simulink model "Robo_Bipede_Contato"  (R2020a)
settings: Solver=ode15s  StartTime=0.0  StopTime=ts  MaxStep=1e-4  RelTol=1e-4  AbsTol=1e-5  EnableMultiTasking=on
model workspace: external: MATLAB File C:\Users\LUIS IZQUIERDO C\Desktop\PROGRAMAS TESE\13. ROBO BIPEDE SIMSCAPE COM CONTATO\Model_Params_Contato.m (data not in the file)
values from neighbouring files (symbols this model uses):
  CoG_y = 0.091733    [Model_Params_Contato.m]
  height_plane = 0.025    [Model_Params_Contato.m]
  m_esfera = 1    [Model_Params_Contato.m]
  plane_height = height_plane    (= 0.025)    [Model_Params_Contato.m]
  plane_length = 50    [Model_Params_Contato.m]
  plane_width = 3    [Model_Params_Contato.m]
  velocidade = 3    [Model_Params_Contato.m]
undefined symbols (not defined in the file or in its folder): COXA, HAT, PE, PERNA, X, Y, Z
libraries: nesl_utility x70, sm_lib x61, simulink_extras x2, simulink x1
(part 2 of 2)

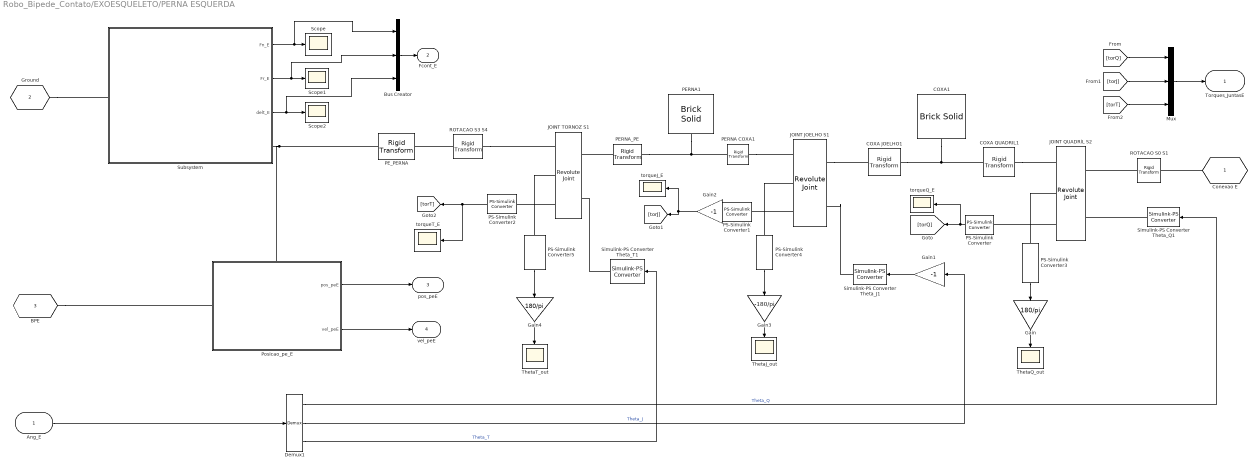
== system Robo_Bipede_Contato/EXOESQUELETO/PERNA ESQUERDA ==
  Ang_E : Inport
  Bus Creator : BusCreator  Inputs=3
  COXA JOELHO1 : sm_lib/Frames and Transforms/Rigid Transform  TranslationMethod=StandardAxis  TranslationStandardOffset=COXA.Comprimento/2  TranslationLengthUnit=m  TranslationStandardAxis=+X  TranslationCartesianOffset=[0 0 0]  TranslationROffset=0  TranslationROffsetUnits=m  TranslationZOffset=0  TranslationZOffsetUnits=m  TranslationThetaOffset=0  TranslationThetaOffsetUnits=deg  RotationMethod=None  RotationAngleUnits=deg  RotationStandardAxis=+Z  RotationAngle=0.0  RotationArbitraryAxis=[0 0 1]  FollAlignAxisA=+X  BaseAlignAxisA=+Y  FollAlignAxisB=+Y  BaseAlignAxisB=+Z  RotationSequenceAxes=FollowerAxes  RotationSequence=XYX  RotationSequenceAngles=[0 0 0]  RotationSequenceAnglesUnits=deg  RotationMatrix=[1 0 0; 0 1 0; 0 0 1]
  COXA QUADRIL1 : sm_lib/Frames and Transforms/Rigid Transform  TranslationMethod=StandardAxis  TranslationStandardOffset=COXA.Comprimento/2  TranslationLengthUnit=m  TranslationStandardAxis=-X  TranslationCartesianOffset=[0 0 0]  TranslationROffset=0  TranslationROffsetUnits=m  TranslationZOffset=0  TranslationZOffsetUnits=m  TranslationThetaOffset=0  TranslationThetaOffsetUnits=deg  RotationMethod=None  RotationAngleUnits=deg  RotationStandardAxis=+Z  RotationAngle=0.0  RotationArbitraryAxis=[0 0 1]  FollAlignAxisA=+X  BaseAlignAxisA=+Y  FollAlignAxisB=+Y  BaseAlignAxisB=+Z  RotationSequenceAxes=FollowerAxes  RotationSequence=XYX  RotationSequenceAngles=[0 0 0]  RotationSequenceAnglesUnits=deg  RotationMatrix=[1 0 0; 0 1 0; 0 0 1]
  COXA1 : sm_lib/Body Elements/Brick Solid  GraphicAmbientColor=[0.15 0.15 0.15 1.0]  BasedOnType=Density  BrickDimensions="[COXA.Comprimento,  COXA.Profundidade,  COXA.Largura]"  BrickDimensionUnits=m  CenterOfMass=[0 0 0]  CenterOfMassUnits=m  GraphicDiffuseColor=cor_coxa  Density=rho_ABS  DensityUnits=kg/m^3  DoExposeReferenceFrame=on  GraphicEmissiveColor=[0.0 0.0 0.0 1.0]  ExportEntireGeometry=off  SerializedFrames=<Frames/>  MarkerShape=Sphere  MarkerSize=10  GraphicType=FromGeometry  InertiaType=CalculateFromGeometry  Mass=1  MassUnits=kg  MomentsOfInertia=[1 1 1]  MomentsOfInertiaUnits=kg*m^2  GraphicOpacity=1.0  ProductsOfInertia=[0 0 0]  ProductsOfInertiaUnits=kg*m^2  GraphicShininess=75  GraphicSpecularColor=[0.5 0.5 0.5 1.0]  GraphicVisPropType=SimpleVisualProperties
  Demux1 : Demux  Outputs=3
  Gain : Gain  Gain=180/pi
  Gain1 : Gain  Gain=-1
  Gain2 : Gain  Gain=-1
  Gain3 : Gain  Gain=-180/pi
  Gain4 : Gain  Gain=180/pi
  JOINT JOELHO S1 : sm_lib/Joints/Revolute Joint  JointMode=Normal  SenseConstraintForce=off  SenseConstraintForceX=off  SenseConstraintForceY=off  SenseConstraintForceZ=off  SenseConstraintTorque=off  SenseConstraintTorqueX=off  SenseConstraintTorqueY=off  SenseConstraintTorqueZ=off  SenseTotalForce=off  SenseTotalForceX=off  SenseTotalForceY=off  SenseTotalForceZ=off  SenseTotalTorque=off  SenseTotalTorqueX=off  SenseTotalTorqueY=off  SenseTotalTorqueZ=off  CompositeWrenchDir=FollowerOnBase  CompositeWrenchFrame=BaseFrame  EquilibriumPosition=0  EquilibriumPositionUnits=rad  SpringStiffness=0  SpringStiffnessUnits=N*m/rad  DampingCoefficient=Damping_junta  DampingCoefficientUnits=N*m/(rad/s)  TorqueActuationMode=ComputedTorque  MotionActuationMode=InputMotion  SensePosition=on  SenseVelocity=off  SenseAcceleration=off  SenseTorqueForce=on  SenseLowerLimitTorqueForce=off  SenseUpperLimitTorqueForce=off  LowerLimitSpecify=off  LowerLimitBound=-90  LowerLimitBoundUnits=deg  LowerLimitStiffness=1e4  LowerLimitStiffnessUnits=N*m/deg  LowerLimitDamping=10  LowerLimitDampingUnits=N*m/(deg/s)  LowerLimitTransitionRegionWidth=0.1  LowerLimitTransitionRegionWidthUnits=deg  UpperLimitSpecify=off  UpperLimitBound=90  UpperLimitBoundUnits=deg  UpperLimitStiffness=1e4  UpperLimitStiffnessUnits=N*m/deg  UpperLimitDamping=10  UpperLimitDampingUnits=N*m/(deg/s)  UpperLimitTransitionRegionWidth=0.1  UpperLimitTransitionRegionWidthUnits=deg  PositionTargetSpecify=on  PositionTargetPriority=High  PositionTargetValue=thetaJ_E0  PositionTargetValueUnits=rad  VelocityTargetSpecify=off  VelocityTargetPriority=High  VelocityTargetValue=0  VelocityTargetValueUnits=deg/s
  JOINT QUADRlL S2 : sm_lib/Joints/Revolute Joint  JointMode=Normal  SenseConstraintForce=off  SenseConstraintForceX=off  SenseConstraintForceY=off  SenseConstraintForceZ=off  SenseConstraintTorque=off  SenseConstraintTorqueX=off  SenseConstraintTorqueY=off  SenseConstraintTorqueZ=off  SenseTotalForce=off  SenseTotalForceX=off  SenseTotalForceY=off  SenseTotalForceZ=off  SenseTotalTorque=off  SenseTotalTorqueX=off  SenseTotalTorqueY=off  SenseTotalTorqueZ=off  CompositeWrenchDir=FollowerOnBase  CompositeWrenchFrame=BaseFrame  EquilibriumPosition=0  EquilibriumPositionUnits=rad  SpringStiffness=0  SpringStiffnessUnits=N*m/rad  DampingCoefficient=Damping_junta  DampingCoefficientUnits=N*m/(rad/s)  TorqueActuationMode=ComputedTorque  MotionActuationMode=InputMotion  SensePosition=on  SenseVelocity=off  SenseAcceleration=off  SenseTorqueForce=on  SenseLowerLimitTorqueForce=off  SenseUpperLimitTorqueForce=off  LowerLimitSpecify=off  LowerLimitBound=-90  LowerLimitBoundUnits=deg  LowerLimitStiffness=1e4  LowerLimitStiffnessUnits=N*m/deg  LowerLimitDamping=10  LowerLimitDampingUnits=N*m/(deg/s)  LowerLimitTransitionRegionWidth=0.1  LowerLimitTransitionRegionWidthUnits=deg  UpperLimitSpecify=off  UpperLimitBound=90  UpperLimitBoundUnits=deg  UpperLimitStiffness=1e4  UpperLimitStiffnessUnits=N*m/deg  UpperLimitDamping=10  UpperLimitDampingUnits=N*m/(deg/s)  UpperLimitTransitionRegionWidth=0.1  UpperLimitTransitionRegionWidthUnits=deg  PositionTargetSpecify=on  PositionTargetPriority=High  PositionTargetValue=thetaQ_E0  PositionTargetValueUnits=rad  VelocityTargetSpecify=off  VelocityTargetPriority=High  VelocityTargetValue=0  VelocityTargetValueUnits=deg/s
  JOINT TORNOZ S1 : sm_lib/Joints/Revolute Joint  JointMode=Normal  SenseConstraintForce=off  SenseConstraintForceX=off  SenseConstraintForceY=off  SenseConstraintForceZ=off  SenseConstraintTorque=off  SenseConstraintTorqueX=off  SenseConstraintTorqueY=off  SenseConstraintTorqueZ=off  SenseTotalForce=off  SenseTotalForceX=off  SenseTotalForceY=off  SenseTotalForceZ=off  SenseTotalTorque=off  SenseTotalTorqueX=off  SenseTotalTorqueY=off  SenseTotalTorqueZ=off  CompositeWrenchDir=FollowerOnBase  CompositeWrenchFrame=BaseFrame  EquilibriumPosition=0  EquilibriumPositionUnits=rad  SpringStiffness=0  SpringStiffnessUnits=N*m/rad  DampingCoefficient=Damping_junta  DampingCoefficientUnits=N*m/(rad/s)  TorqueActuationMode=ComputedTorque  MotionActuationMode=InputMotion  SensePosition=on  SenseVelocity=off  SenseAcceleration=off  SenseTorqueForce=on  SenseLowerLimitTorqueForce=off  SenseUpperLimitTorqueForce=off  LowerLimitSpecify=off  LowerLimitBound=-90  LowerLimitBoundUnits=deg  LowerLimitStiffness=1e4  LowerLimitStiffnessUnits=N*m/deg  LowerLimitDamping=10  LowerLimitDampingUnits=N*m/(deg/s)  LowerLimitTransitionRegionWidth=0.1  LowerLimitTransitionRegionWidthUnits=deg  UpperLimitSpecify=off  UpperLimitBound=90  UpperLimitBoundUnits=deg  UpperLimitStiffness=1e4  UpperLimitStiffnessUnits=N*m/deg  UpperLimitDamping=10  UpperLimitDampingUnits=N*m/(deg/s)  UpperLimitTransitionRegionWidth=0.1  UpperLimitTransitionRegionWidthUnits=deg  PositionTargetSpecify=on  PositionTargetPriority=High  PositionTargetValue=thetaT_E0  PositionTargetValueUnits=rad  VelocityTargetSpecify=off  VelocityTargetPriority=High  VelocityTargetValue=0  VelocityTargetValueUnits=deg/s
  Mux : Mux  Inputs=3
  PERNA COXA1 : sm_lib/Frames and Transforms/Rigid Transform  TranslationMethod=StandardAxis  TranslationStandardOffset=PERNA.Comprimento/2  TranslationLengthUnit=m  TranslationStandardAxis=-X  TranslationCartesianOffset=[0 0 0]  TranslationROffset=0  TranslationROffsetUnits=m  TranslationZOffset=0  TranslationZOffsetUnits=m  TranslationThetaOffset=0  TranslationThetaOffsetUnits=deg  RotationMethod=None  RotationAngleUnits=deg  RotationStandardAxis=+Z  RotationAngle=0.0  RotationArbitraryAxis=[0 0 1]  FollAlignAxisA=+X  BaseAlignAxisA=+Y  FollAlignAxisB=+Y  BaseAlignAxisB=+Z  RotationSequenceAxes=FollowerAxes  RotationSequence=XYX  RotationSequenceAngles=[0 0 0]  RotationSequenceAnglesUnits=deg  RotationMatrix=[1 0 0; 0 1 0; 0 0 1]
  PERNA1 : sm_lib/Body Elements/Brick Solid  GraphicAmbientColor=[0.15 0.15 0.15 1.0]  BasedOnType=Density  BrickDimensions=[PERNA.Comprimento, PERNA.Profundidade, PERNA.Largura]  BrickDimensionUnits=m  CenterOfMass=[0 0 0]  CenterOfMassUnits=m  GraphicDiffuseColor=cor_perna  Density=rho_ABS  DensityUnits=kg/m^3  DoExposeReferenceFrame=on  GraphicEmissiveColor=[0.0 0.0 0.0 1.0]  ExportEntireGeometry=off  SerializedFrames=<Frames/>  MarkerShape=Sphere  MarkerSize=10  GraphicType=FromGeometry  InertiaType=CalculateFromGeometry  Mass=1  MassUnits=kg  MomentsOfInertia=[1 1 1]  MomentsOfInertiaUnits=kg*m^2  GraphicOpacity=1.0  ProductsOfInertia=[0 0 0]  ProductsOfInertiaUnits=kg*m^2  GraphicShininess=75  GraphicSpecularColor=[0.5 0.5 0.5 1.0]  GraphicVisPropType=SimpleVisualProperties
  PERNA_PE : sm_lib/Frames and Transforms/Rigid Transform  TranslationMethod=Cartesian  TranslationStandardOffset=0  TranslationLengthUnit=m  TranslationStandardAxis=+Z  TranslationCartesianOffset=[PERNA.Comprimento/2, -PERNA.Profundidade/2, 0]  TranslationROffset=0  TranslationROffsetUnits=m  TranslationZOffset=0  TranslationZOffsetUnits=m  TranslationThetaOffset=0  TranslationThetaOffsetUnits=deg  RotationMethod=None  RotationAngleUnits=deg  RotationStandardAxis=+Z  RotationAngle=0.0  RotationArbitraryAxis=[0 0 1]  FollAlignAxisA=+X  BaseAlignAxisA=+Y  FollAlignAxisB=+Y  BaseAlignAxisB=+Z  RotationSequenceAxes=FollowerAxes  RotationSequence=XYX  RotationSequenceAngles=[0 0 0]  RotationSequenceAnglesUnits=deg  RotationMatrix=[1 0 0; 0 1 0; 0 0 1]
  PE_PERNA : sm_lib/Frames and Transforms/Rigid Transform  TranslationMethod=Cartesian  TranslationStandardOffset=0  TranslationLengthUnit=m  TranslationStandardAxis=+Z  TranslationCartesianOffset=[-PE.Comprimento/2, 0, 0]  TranslationROffset=0  TranslationROffsetUnits=m  TranslationZOffset=0  TranslationZOffsetUnits=m  TranslationThetaOffset=0  TranslationThetaOffsetUnits=deg  RotationMethod=None  RotationAngleUnits=deg  RotationStandardAxis=+Z  RotationAngle=0.0  RotationArbitraryAxis=[0 0 1]  FollAlignAxisA=+X  BaseAlignAxisA=+Y  FollAlignAxisB=+Y  BaseAlignAxisB=+Z  RotationSequenceAxes=FollowerAxes  RotationSequence=XYX  RotationSequenceAngles=[0 0 0]  RotationSequenceAnglesUnits=deg  RotationMatrix=[1 0 0; 0 1 0; 0 0 1]
  PS-Simulink Converter : nesl_utility/PS-Simulink Converter  PhysicalDomain=network_engine_domain  SubClassName=ps_output  LeftPortType=input  RightPortType=output  PseudoPeriodic=off  Frequencies=[]  Unit=N*m  AffineConversion=off
  PS-Simulink Converter1 : nesl_utility/PS-Simulink Converter  PhysicalDomain=network_engine_domain  SubClassName=ps_output  LeftPortType=input  RightPortType=output  PseudoPeriodic=off  Frequencies=[]  Unit=N*m  AffineConversion=off
  PS-Simulink Converter2 : nesl_utility/PS-Simulink Converter  PhysicalDomain=network_engine_domain  SubClassName=ps_output  LeftPortType=input  RightPortType=output  PseudoPeriodic=off  Frequencies=[]  Unit=N*m  AffineConversion=off
  PS-Simulink Converter3 : nesl_utility/PS-Simulink Converter  PhysicalDomain=network_engine_domain  SubClassName=ps_output  LeftPortType=input  RightPortType=output  PseudoPeriodic=off  Frequencies=[]  Unit=1  AffineConversion=off
  PS-Simulink Converter4 : nesl_utility/PS-Simulink Converter  PhysicalDomain=network_engine_domain  SubClassName=ps_output  LeftPortType=input  RightPortType=output  PseudoPeriodic=off  Frequencies=[]  Unit=1  AffineConversion=off
  PS-Simulink Converter5 : nesl_utility/PS-Simulink Converter  PhysicalDomain=network_engine_domain  SubClassName=ps_output  LeftPortType=input  RightPortType=output  PseudoPeriodic=off  Frequencies=[]  Unit=1  AffineConversion=off
  Posicao_pe_E : Subsystem
      settings: PortSchema="{\"entries\":[{\"content\":{\"sides\":[{\"content\":{\"connectorIds\":[\"LConn1\"]},\"type\":\"ConnectorPlacement.EquallySpacedRectSide\",\"uuid\":\"d1ecfdf8-7ebe-4af1-bf63-6510536b3168\"},{\"content\":{\"connectorIds\":[\"Out1\",\"Out2\"],\"side\":\"RIGHT\"},\"type\":\"ConnectorPlacement.EquallySpacedRectSide\",\"uuid\":\"ea2203bb-aad8-4cc6-b714-1d05e8985fb0\"},{\"content\":{\"connectorIds\":[\"LConn2\"],\"side\":\"TOP\"},\"type\":\"ConnectorPlacement.EquallySpacedRectSide\",\"uuid\":\"9c93785d-a169-4ae6-a4ad-27289c508aaf\"}]},\"type\":\"ConnectorPlacement.EquallySpacedConnector\",\"uuid\":\"0aa9c047-7b9e-44d9-9c0d-089578f3a65a\"}],\"packageUris\":[\"http://schema.mathworks.com/mf0/Connector/19700101\"],\"version\":\"1.0\"}"
  ROTACAO S0 S1 : sm_lib/Frames and Transforms/Rigid Transform  TranslationMethod=None  TranslationStandardOffset=0  TranslationLengthUnit=m  TranslationStandardAxis=+Z  TranslationCartesianOffset=[0 0 0]  TranslationROffset=0  TranslationROffsetUnits=m  TranslationZOffset=0  TranslationZOffsetUnits=m  TranslationThetaOffset=0  TranslationThetaOffsetUnits=deg  RotationMethod=StandardAxis  RotationAngleUnits=deg  RotationStandardAxis=+Z  RotationAngle=-90  RotationArbitraryAxis=[0 0 1]  FollAlignAxisA=+X  BaseAlignAxisA=+Y  FollAlignAxisB=+Y  BaseAlignAxisB=+Z  RotationSequenceAxes=FollowerAxes  RotationSequence=XYX  RotationSequenceAngles=[0 0 0]  RotationSequenceAnglesUnits=deg  RotationMatrix=[1 0 0; 0 1 0; 0 0 1]
  ROTACAO S3 S4 : sm_lib/Frames and Transforms/Rigid Transform  TranslationMethod=None  TranslationStandardOffset=0  TranslationLengthUnit=m  TranslationStandardAxis=+Z  TranslationCartesianOffset=[0 0 0]  TranslationROffset=0  TranslationROffsetUnits=m  TranslationZOffset=0  TranslationZOffsetUnits=m  TranslationThetaOffset=0  TranslationThetaOffsetUnits=deg  RotationMethod=StandardAxis  RotationAngleUnits=deg  RotationStandardAxis=+Z  RotationAngle=90  RotationArbitraryAxis=[0 0 1]  FollAlignAxisA=+X  BaseAlignAxisA=+Y  FollAlignAxisB=+Y  BaseAlignAxisB=+Z  RotationSequenceAxes=FollowerAxes  RotationSequence=XYX  RotationSequenceAngles=[0 0 0]  RotationSequenceAnglesUnits=deg  RotationMatrix=[1 0 0; 0 1 0; 0 0 1]
  Scope : Scope
  Scope1 : Scope
  Scope2 : Scope
  Simulink-PS Converter Theta_J1 : nesl_utility/Simulink-PS Converter  PhysicalDomain=network_engine_domain  SubClassName=ps_input  LeftPortType=input  RightPortType=output  PseudoPeriodic=off  Frequencies=[]  NoiseDistribution=none  NoiseParameters=[]  Unit=rad  AffineConversion=off  FilteringAndDerivatives=filter  SimscapeFilterOrder=2  InputFilterTimeConstant=motion_time_constant  UdotUserProvided=0
  Simulink-PS Converter Theta_Q1 : nesl_utility/Simulink-PS Converter  PhysicalDomain=network_engine_domain  SubClassName=ps_input  LeftPortType=input  RightPortType=output  PseudoPeriodic=off  Frequencies=[]  NoiseDistribution=none  NoiseParameters=[]  Unit=rad  AffineConversion=off  FilteringAndDerivatives=filter  SimscapeFilterOrder=2  InputFilterTimeConstant=motion_time_constant  UdotUserProvided=0
  Simulink-PS Converter Theta_T1 : nesl_utility/Simulink-PS Converter  PhysicalDomain=network_engine_domain  SubClassName=ps_input  LeftPortType=input  RightPortType=output  PseudoPeriodic=off  Frequencies=[]  NoiseDistribution=none  NoiseParameters=[]  Unit=rad  AffineConversion=off  FilteringAndDerivatives=filter  SimscapeFilterOrder=2  InputFilterTimeConstant=motion_time_constant  UdotUserProvided=0
  Subsystem : Subsystem
  ThetaJ_out : Scope
  ThetaQ_out : Scope
  ThetaT_out : Scope
  torqueJ_E : Scope
  torqueQ_E : Scope
  torqueT_E : Scope
  Conexao E : PMIOPort  Side=Left
  Ground : PMIOPort  Port=2  Side=Left
  BPE : PMIOPort  Port=3  Side=Left
  "Torques_JuntasE " : Outport  VectorParamsAs1DForOutWhenUnconnected=off
  Fcont_E : Outport  Port=2
  pos_peE : Outport  Port=3
  vel_peE : Outport  Port=4
  wires:
  Gain2/1 -> torqueJ_E/1, [torJ]
  [torQ] -> Mux/1
  Mux/1 -> "Torques_JuntasE "/1
  [torT] -> Mux/3
  PS-Simulink Converter1/1 -> Gain2/1
  Ang_E/1 -> Demux1/1
  PS-Simulink Converter2/1 -> torqueT_E/1, [torT]
  PS-Simulink Converter/1 -> torqueQ_E/1, [torQ]
  Gain1/1 -> Simulink-PS Converter Theta_J1/1
  Demux1/1 -> Simulink-PS Converter Theta_Q1/1  "Theta_Q"
  Demux1/2 -> Gain1/1  "Theta_J"
  Demux1/3 -> Simulink-PS Converter Theta_T1/1  "Theta_T"
  [torJ] -> Mux/2
  Gain/1 -> ThetaQ_out/1
  PS-Simulink Converter3/1 -> Gain/1
  Gain3/1 -> ThetaJ_out/1
  PS-Simulink Converter4/1 -> Gain3/1
  PS-Simulink Converter5/1 -> Gain4/1
  Gain4/1 -> ThetaT_out/1
  Subsystem/3(delt_E) -> Bus Creator/3, Scope2/1
  Subsystem/2(Fr_E) -> Bus Creator/2, Scope1/1
  Subsystem/1(Fn_E) -> Bus Creator/1, Scope/1
  Bus Creator/1 -> Fcont_E/1
  Posicao_pe_E/1(pos_peE) -> pos_peE/1
  Posicao_pe_E/2(vel_peE) -> vel_peE/1
  connections:
  ROTACAO S3 S4/LConn1 -- JOINT TORNOZ S1/RConn1
  COXA JOELHO1/LConn1 -- COXA1/RConn1 -- COXA QUADRIL1/LConn1
  PERNA1/RConn1 -- PERNA COXA1/LConn1 -- PERNA_PE/LConn1
  ROTACAO S3 S4/RConn1 -- PE_PERNA/RConn1
  Simulink-PS Converter Theta_T1/RConn1 -- JOINT TORNOZ S1/LConn2
  PERNA COXA1/RConn1 -- JOINT JOELHO S1/RConn1
  Simulink-PS Converter Theta_Q1/RConn1 -- JOINT QUADRlL S2/LConn2
  JOINT JOELHO S1/LConn1 -- COXA JOELHO1/RConn1
  Simulink-PS Converter Theta_J1/RConn1 -- JOINT JOELHO S1/LConn2
  ROTACAO S0 S1/RConn1 -- JOINT QUADRlL S2/LConn1
  COXA QUADRIL1/RConn1 -- JOINT QUADRlL S2/RConn1
  Conexao E/RConn1 -- ROTACAO S0 S1/LConn1
  JOINT QUADRlL S2/RConn2 -- PS-Simulink Converter3/LConn1
  JOINT QUADRlL S2/RConn3 -- PS-Simulink Converter/LConn1
  JOINT JOELHO S1/RConn2 -- PS-Simulink Converter4/LConn1
  JOINT JOELHO S1/RConn3 -- PS-Simulink Converter1/LConn1
  JOINT TORNOZ S1/RConn2 -- PS-Simulink Converter5/LConn1
  JOINT TORNOZ S1/RConn3 -- PS-Simulink Converter2/LConn1
  PERNA_PE/RConn1 -- JOINT TORNOZ S1/LConn1
  Ground/RConn1 -- Subsystem/LConn1
  PE_PERNA/LConn1 -- Posicao_pe_E/LConn2 -- Subsystem/RConn1
  BPE/RConn1 -- Posicao_pe_E/LConn1

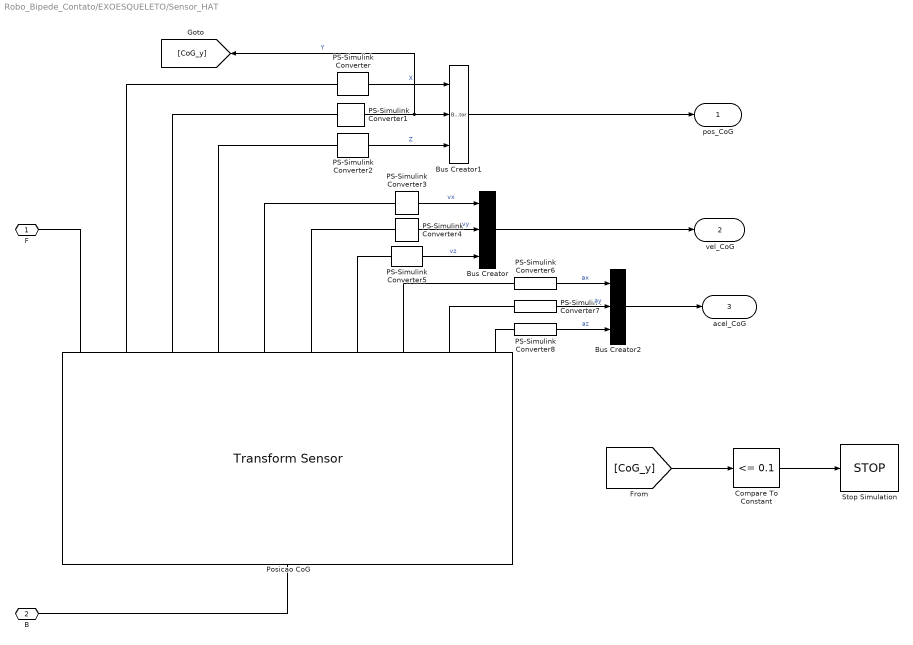
== system Robo_Bipede_Contato/EXOESQUELETO/Sensor_HAT ==
  Bus Creator : BusCreator  Inputs=3
  Bus Creator1 : BusCreator  Inputs=3
  Bus Creator2 : BusCreator  Inputs=3
  Compare To Constant : simulink/Logic and Bit Operations/Compare To Constant  relop=<=  const=0.1  OutDataTypeStr=boolean
  PS-Simulink Converter : nesl_utility/PS-Simulink Converter  PhysicalDomain=network_engine_domain  SubClassName=ps_output  LeftPortType=input  RightPortType=output  PseudoPeriodic=off  Frequencies=[]  Unit=m  AffineConversion=off
  PS-Simulink Converter1 : nesl_utility/PS-Simulink Converter  PhysicalDomain=network_engine_domain  SubClassName=ps_output  LeftPortType=input  RightPortType=output  PseudoPeriodic=off  Frequencies=[]  Unit=m  AffineConversion=off
  PS-Simulink Converter2 : nesl_utility/PS-Simulink Converter  PhysicalDomain=network_engine_domain  SubClassName=ps_output  LeftPortType=input  RightPortType=output  PseudoPeriodic=off  Frequencies=[]  Unit=m  AffineConversion=off
  PS-Simulink Converter3 : nesl_utility/PS-Simulink Converter  PhysicalDomain=network_engine_domain  SubClassName=ps_output  LeftPortType=input  RightPortType=output  PseudoPeriodic=off  Frequencies=[]  Unit=m/s  AffineConversion=off
  PS-Simulink Converter4 : nesl_utility/PS-Simulink Converter  PhysicalDomain=network_engine_domain  SubClassName=ps_output  LeftPortType=input  RightPortType=output  PseudoPeriodic=off  Frequencies=[]  Unit=m/s  AffineConversion=off
  PS-Simulink Converter5 : nesl_utility/PS-Simulink Converter  PhysicalDomain=network_engine_domain  SubClassName=ps_output  LeftPortType=input  RightPortType=output  PseudoPeriodic=off  Frequencies=[]  Unit=m/s  AffineConversion=off
  PS-Simulink Converter6 : nesl_utility/PS-Simulink Converter  PhysicalDomain=network_engine_domain  SubClassName=ps_output  LeftPortType=input  RightPortType=output  PseudoPeriodic=off  Frequencies=[]  Unit=inherit  AffineConversion=off
  PS-Simulink Converter7 : nesl_utility/PS-Simulink Converter  PhysicalDomain=network_engine_domain  SubClassName=ps_output  LeftPortType=input  RightPortType=output  PseudoPeriodic=off  Frequencies=[]  Unit=inherit  AffineConversion=off
  PS-Simulink Converter8 : nesl_utility/PS-Simulink Converter  PhysicalDomain=network_engine_domain  SubClassName=ps_output  LeftPortType=input  RightPortType=output  PseudoPeriodic=off  Frequencies=[]  Unit=inherit  AffineConversion=off
  Posicao CoG : sm_lib/Frames and Transforms/Transform Sensor  MeasurementFrame=Base  SenseAngle=off  SenseAxis=off  SenseAngle1=off  SenseAngle2=off  SenseAngle3=off  SenseQ=off  SenseR=off  SenseOmegaX=off  SenseOmegaY=off  SenseOmegaZ=off  SenseOmega1=off  SenseOmega2=off  SenseOmega3=off  SenseQDot=off  SenseRDot=off  SenseAlphaX=off  SenseAlphaY=off  SenseAlphaZ=off  SenseAlpha1=off  SenseAlpha2=off  SenseAlpha3=off  SenseQDDot=off  SenseRDDot=off  SenseX=on  SenseY=on  SenseZ=on  SenseRad=off  SenseAzim=off  SenseDist=off  SenseInc=off  SenseXDot=on  SenseYDot=on  SenseZDot=on  SenseRadDot=off  SenseAzimDot=off  SenseDistDot=off  SenseIncDot=off  SenseXDDot=on  SenseYDDot=on  SenseZDDot=on  SenseRadDDot=off  SenseAzimDDot=off  SenseDistDDot=off  SenseIncDDot=off
  Stop Simulation : Stop
  F : PMIOPort  Side=Left
  B : PMIOPort  Port=2  Side=Right
  pos_CoG : Outport
  vel_CoG : Outport  Port=2
  acel_CoG : Outport  Port=3
  wires:
  Compare To Constant/1 -> Stop Simulation/1
  [CoG_y] -> Compare To Constant/1
  PS-Simulink Converter/1 -> Bus Creator1/1  "X"
  PS-Simulink Converter1/1 -> [CoG_y], Bus Creator1/2  "Y"
  PS-Simulink Converter2/1 -> Bus Creator1/3  "Z"
  PS-Simulink Converter3/1 -> Bus Creator/1  "vx"
  PS-Simulink Converter4/1 -> Bus Creator/2  "vy"
  PS-Simulink Converter5/1 -> Bus Creator/3  "vz"
  PS-Simulink Converter6/1 -> Bus Creator2/1  "ax"
  PS-Simulink Converter7/1 -> Bus Creator2/2  "ay"
  PS-Simulink Converter8/1 -> Bus Creator2/3  "az"
  Bus Creator1/1 -> pos_CoG/1
  Bus Creator/1 -> vel_CoG/1
  Bus Creator2/1 -> acel_CoG/1
  connections:
  PS-Simulink Converter2/LConn1 -- Posicao CoG/RConn4
  PS-Simulink Converter1/LConn1 -- Posicao CoG/RConn3
  Posicao CoG/RConn1 -- F/RConn1
  PS-Simulink Converter/LConn1 -- Posicao CoG/RConn2
  Posicao CoG/LConn1 -- B/RConn1
  PS-Simulink Converter5/LConn1 -- Posicao CoG/RConn7
  PS-Simulink Converter3/LConn1 -- Posicao CoG/RConn5
  PS-Simulink Converter4/LConn1 -- Posicao CoG/RConn6
  PS-Simulink Converter6/LConn1 -- Posicao CoG/RConn8
  PS-Simulink Converter7/LConn1 -- Posicao CoG/RConn9
  PS-Simulink Converter8/LConn1 -- Posicao CoG/RConn10

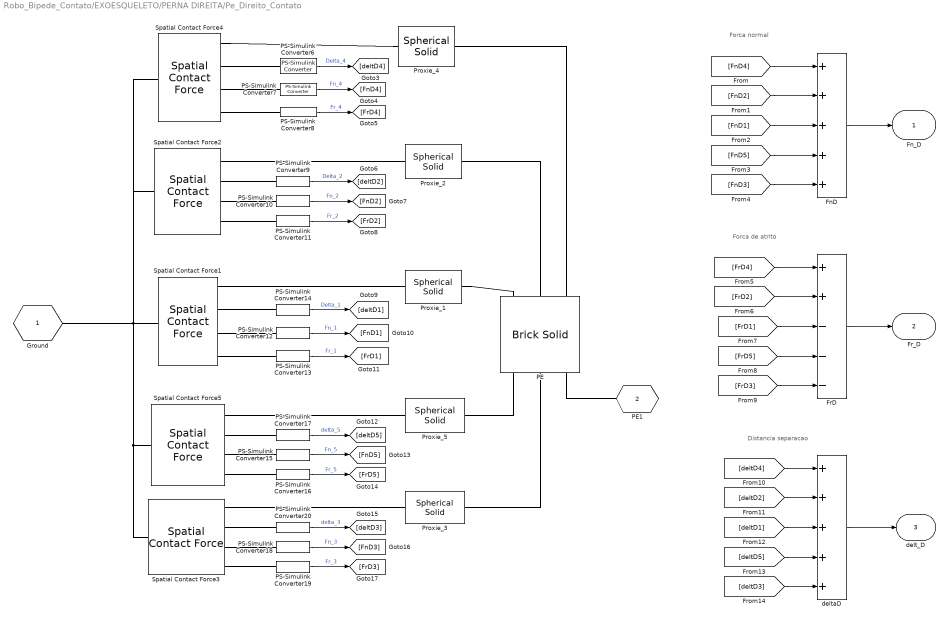
== system Robo_Bipede_Contato/EXOESQUELETO/PERNA DIREITA/Pe_Direito_Contato ==
  note: Distancia separacao
  note: Forca de atrito
  note: Forca normal
  FnD : Sum  Inputs=+++++
  FrD : Sum  Inputs=++---
  PE : sm_lib/Body Elements/Brick Solid  GraphicAmbientColor=[0.15 0.15 0.15 1.0]  BasedOnType=Density  BrickDimensions=[PE.Comprimento, PE.Profundidade, PE.Largura ]  BrickDimensionUnits=m  CenterOfMass=[0 0 0]  CenterOfMassUnits=m  GraphicDiffuseColor=cor_pe  Density=rho_ABS  DensityUnits=kg/m^3  DoExposeReferenceFrame=on  GraphicEmissiveColor=[0.0 0.0 0.0 1.0]  ExportEntireGeometry=off  SerializedFrames=<Frames><Frame><Id>Frame1</Id><Value><Name>F1</Name><Origin><Source>GeometricFeature</Source><FeatureName>+z -x curve</FeatureName></Origin><PrimaryAxis><DefinedDirection>+Z</DefinedDirection><Source>ReferenceFrame</Source><SourceDirection>+Z</SourceDirection><FeatureName></FeatureName></PrimaryAxis><SecondaryAxis><DefinedDirection>+X</DefinedDirection><Source>ReferenceFrame</Source><SourceDirection>+X</SourceDirection><FeatureName></FeatureName></SecondaryAxis></Value></Frame><Frame><Id>Frame2</Id><Value><Name>F2</Name><Origin><Source>GeometricFeature</Source><FeatureName>+z +x curve</FeatureName></Origin><PrimaryAxis><DefinedDirection>+Z</DefinedDirection><Source>ReferenceFrame</Source><SourceDirection>+Z</SourceDirection><FeatureName></FeatureName></PrimaryAxis><SecondaryAxis><DefinedDirection>+X</DefinedDirection><Source>ReferenceFrame</Source><SourceDirection>+X</SourceDirection><FeatureName></FeatureName></SecondaryAxis></Value></Frame><Frame><Id>Frame3</Id><Value><Name>F3</Name><Origin><Source>GeometricFeature</Source><FeatureName>-z -x curve</FeatureName></Origin><PrimaryAxis><DefinedDirection>+Z</DefinedDirection><Source>ReferenceFrame</Source><SourceDirection>+Z</SourceDirection><FeatureName></FeatureName></PrimaryAxis><SecondaryAxis><DefinedDirection>+X</DefinedDirection><Source>ReferenceFrame</Source><SourceDirection>+X</SourceDirection><FeatureName></FeatureName></SecondaryAxis></Value></Frame><Frame><Id>Frame4</Id><Value><Name>F4</Name><Origin><Source>GeometricFeature</Source><FeatureName>-z +x curve</FeatureName></Origin><PrimaryAxis><DefinedDirection>+Z</DefinedDirection><Source>ReferenceFrame</Source><SourceDirection>+Z</SourceDirection><FeatureName></FeatureName></PrimaryAxis><SecondaryAxis><DefinedDirection>+X</DefinedDirection><Source>ReferenceFrame</Source><SourceDirection>+X</SourceDirection><FeatureName></FeatureName></SecondaryAxis></Value></Frame><Frame><Id>Frame5</Id><Value><Name>Sup_Pe</Name><Origin><Source>GeometricFeature</Source><FeatureName>+y surface</FeatureName></Origin><PrimaryAxis><DefinedDirection>+Y</DefinedDirection><Source>ReferenceFrame</Source><SourceDirection>+Y</SourceDirection><FeatureName></FeatureName></PrimaryAxis><SecondaryAxis><DefinedDirection>+X</DefinedDirection><Source>ReferenceFrame</Source><SourceDirection>+X</SourceDirection><FeatureName></FeatureName></SecondaryAxis></Value></Frame></Frames>  MarkerShape=Sphere  MarkerSize=10  GraphicType=FromGeometry  InertiaType=CalculateFromGeometry  Mass=1  MassUnits=kg  MomentsOfInertia=[1 1 1]  MomentsOfInertiaUnits=kg*m^2  GraphicOpacity=1.0  ProductsOfInertia=[0 0 0]  ProductsOfInertiaUnits=kg*m^2  GraphicShininess=75  GraphicSpecularColor=[0.5 0.5 0.5 1.0]  GraphicVisPropType=SimpleVisualProperties
  PS-Simulink Converter{6..20} (15 alike) : nesl_utility/PS-Simulink Converter  PhysicalDomain=network_engine_domain  SubClassName=ps_output  LeftPortType=input  RightPortType=output  PseudoPeriodic=off  Frequencies=[]  Unit=inherit  AffineConversion=off
  Proxie_{1..5} (5 alike) : sm_lib/Body Elements/Spherical Solid  GraphicAmbientColor=[0.15 0.15 0.15 1.0]  BasedOnType=Mass  CenterOfMass=[0 0 0]  CenterOfMassUnits=m  GraphicDiffuseColor=[0.5 0.5 0.5]  Density=rho_ABS  DensityUnits=kg/m^3  DoExposeReferenceFrame=on  GraphicEmissiveColor=[0.0 0.0 0.0 1.0]  ExportEntireGeometry=on  SerializedExposedGeometries=<ExposedGeometries><ExposedGeometry><RawGeometryId>entire</RawGeometryId><ExposedGeometryId>G</ExposedGeometryId></ExposedGeometry></ExposedGeometries>  SerializedFrames=<Frames/>  MarkerShape=Sphere  MarkerSize=10  GraphicType=FromGeometry  InertiaType=CalculateFromGeometry  Mass=m_esfera  MassUnits=g  MomentsOfInertia=[1 1 1]  MomentsOfInertiaUnits=kg*m^2  GraphicOpacity=1.0  ProductsOfInertia=[0 0 0]  ProductsOfInertiaUnits=kg*m^2  GraphicShininess=75  GraphicSpecularColor=[0.5 0.5 0.5 1.0]  SphereRadius=PE.Profundidade/2  SphereRadiusUnits=m  GraphicVisPropType=SimpleVisualProperties
  Spatial Contact Force{1..3,5} (4 alike) : sm_lib/Forces and Torques/Spatial Contact Force  CoefficientOfDynamicFriction=mu_k  CoefficientOfStaticFriction=mu_s  NormalDamping=contact_damping  NormalDampingUnits=N/(m/s)  NormalStiffness=contact_stiffness  NormalStiffnessUnits=N/m  FrictionalCriticalVelocity=mu_vth  FrictionalCriticalVelocityUnits=m/s  ZeroCrossDetectContactStartAndEnd=off  SenseFrictionalForceMagnitude=on  SenseNormalForceMagnitude=on  SenseSeparationDistance=on  NormalTransitionRegionWidth=transition_width  NormalTransitionRegionWidthUnits=m  FrictionType=SmoothStickSlip
  Spatial Contact Force4 : sm_lib/Forces and Torques/Spatial Contact Force  CoefficientOfDynamicFriction=mu_k  CoefficientOfStaticFriction=mu_s  NormalDamping=contact_damping  NormalDampingUnits=N/(m/s)  NormalStiffness=contact_stiffness  NormalStiffnessUnits=N/m  FrictionalCriticalVelocity=mu_vth  FrictionalCriticalVelocityUnits=m/s  ZeroCrossDetectContactStartAndEnd=on  SenseFrictionalForceMagnitude=on  SenseNormalForceMagnitude=on  SenseSeparationDistance=on  NormalTransitionRegionWidth=transition_width  NormalTransitionRegionWidthUnits=m  FrictionType=SmoothStickSlip
  deltaD : Sum  Inputs=+++++
  Ground : PMIOPort  Side=Left
  PE1 : PMIOPort  Port=2  Side=Right
  Fn_D : Outport
  Fr_D : Outport  Port=2
  delt_D : Outport  Port=3
  wires:
  PS-Simulink Converter17/1 -> [deltD5]  "delta_5"
  PS-Simulink Converter7/1 -> [FnD4]  "Fn_4"
  PS-Simulink Converter16/1 -> [FrD5]  "Fr_5"
  PS-Simulink Converter15/1 -> [FnD5]  "Fn_5"
  PS-Simulink Converter10/1 -> [FnD2]  "Fn_2"
  PS-Simulink Converter12/1 -> [FnD1]  "Fn_1"
  PS-Simulink Converter13/1 -> [FrD1]  "Fr_1"
  PS-Simulink Converter8/1 -> [FrD4]  "Fr_4"
  PS-Simulink Converter19/1 -> [FrD3]  "Fr_3"
  PS-Simulink Converter9/1 -> [deltD2]  "Delta_2"
  PS-Simulink Converter14/1 -> [deltD1]  "Delta_1"
  PS-Simulink Converter18/1 -> [FnD3]  "Fn_3"
  PS-Simulink Converter6/1 -> [deltD4]  "Delta_4"
  PS-Simulink Converter20/1 -> [deltD3]  "delta_3"
  PS-Simulink Converter11/1 -> [FrD2]  "Fr_2"
  [FnD4] -> FnD/1
  [FnD2] -> FnD/2
  [FnD1] -> FnD/3
  [FnD5] -> FnD/4
  [FnD3] -> FnD/5
  [FrD4] -> FrD/1
  [FrD2] -> FrD/2
  [FrD1] -> FrD/3
  [FrD5] -> FrD/4
  [FrD3] -> FrD/5
  [deltD4] -> deltaD/1
  [deltD2] -> deltaD/2
  [deltD1] -> deltaD/3
  [deltD5] -> deltaD/4
  [deltD3] -> deltaD/5
  FnD/1 -> Fn_D/1
  FrD/1 -> Fr_D/1
  deltaD/1 -> delt_D/1
  connections:
  PS-Simulink Converter17/LConn1 -- Spatial Contact Force5/RConn2
  Proxie_4/RConn1 -- PE/LConn3
  PS-Simulink Converter6/LConn1 -- Spatial Contact Force4/RConn2
  Proxie_3/RConn1 -- PE/RConn2
  Proxie_1/RConn1 -- PE/LConn1
  PS-Simulink Converter19/LConn1 -- Spatial Contact Force3/RConn4
  PS-Simulink Converter8/LConn1 -- Spatial Contact Force4/RConn4
  Proxie_2/RConn1 -- PE/LConn2
  Spatial Contact Force1/RConn1 -- Proxie_1/LConn1
  PS-Simulink Converter10/LConn1 -- Spatial Contact Force2/RConn3
  PS-Simulink Converter12/LConn1 -- Spatial Contact Force1/RConn3
  Proxie_5/RConn1 -- PE/RConn1
  Proxie_5/LConn1 -- Spatial Contact Force5/RConn1
  Spatial Contact Force3/RConn1 -- Proxie_3/LConn1
  PS-Simulink Converter18/LConn1 -- Spatial Contact Force3/RConn3
  Spatial Contact Force5/LConn1 -- Spatial Contact Force4/LConn1 -- Spatial Contact Force2/LConn1 -- Ground/RConn1 -- Spatial Contact Force1/LConn1 -- Spatial Contact Force3/LConn1
  Spatial Contact Force2/RConn1 -- Proxie_2/LConn1
  PS-Simulink Converter20/LConn1 -- Spatial Contact Force3/RConn2
  PS-Simulink Converter7/LConn1 -- Spatial Contact Force4/RConn3
  Spatial Contact Force5/RConn3 -- PS-Simulink Converter15/LConn1
  Spatial Contact Force4/RConn1 -- Proxie_4/LConn1
  PS-Simulink Converter9/LConn1 -- Spatial Contact Force2/RConn2
  Spatial Contact Force5/RConn4 -- PS-Simulink Converter16/LConn1
  PS-Simulink Converter14/LConn1 -- Spatial Contact Force1/RConn2
  PS-Simulink Converter13/LConn1 -- Spatial Contact Force1/RConn4
  PS-Simulink Converter11/LConn1 -- Spatial Contact Force2/RConn4
  PE1/RConn1 -- PE/RConn3

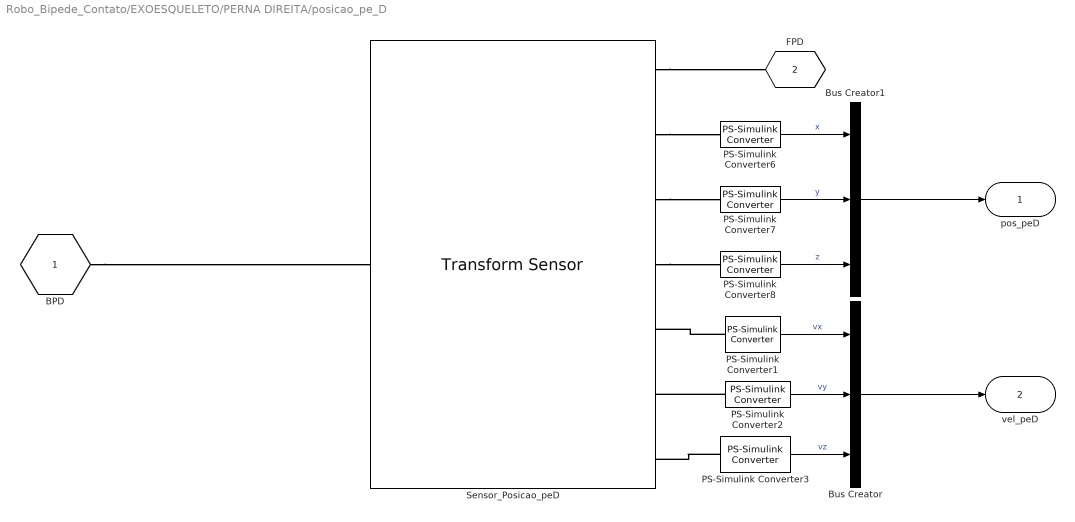
== system Robo_Bipede_Contato/EXOESQUELETO/PERNA DIREITA/posicao_pe_D ==
  Bus Creator : BusCreator  Inputs=3
  Bus Creator1 : BusCreator  Inputs=3
  PS-Simulink Converter1 : nesl_utility/PS-Simulink Converter  PhysicalDomain=network_engine_domain  SubClassName=ps_output  LeftPortType=input  RightPortType=output  PseudoPeriodic=off  Frequencies=[]  Unit=m/s  AffineConversion=off
  PS-Simulink Converter2 : nesl_utility/PS-Simulink Converter  PhysicalDomain=network_engine_domain  SubClassName=ps_output  LeftPortType=input  RightPortType=output  PseudoPeriodic=off  Frequencies=[]  Unit=m/s  AffineConversion=off
  PS-Simulink Converter3 : nesl_utility/PS-Simulink Converter  PhysicalDomain=network_engine_domain  SubClassName=ps_output  LeftPortType=input  RightPortType=output  PseudoPeriodic=off  Frequencies=[]  Unit=m/s  AffineConversion=off
  PS-Simulink Converter6 : nesl_utility/PS-Simulink Converter  PhysicalDomain=network_engine_domain  SubClassName=ps_output  LeftPortType=input  RightPortType=output  PseudoPeriodic=off  Frequencies=[]  Unit=m  AffineConversion=off
  PS-Simulink Converter7 : nesl_utility/PS-Simulink Converter  PhysicalDomain=network_engine_domain  SubClassName=ps_output  LeftPortType=input  RightPortType=output  PseudoPeriodic=off  Frequencies=[]  Unit=m  AffineConversion=off
  PS-Simulink Converter8 : nesl_utility/PS-Simulink Converter  PhysicalDomain=network_engine_domain  SubClassName=ps_output  LeftPortType=input  RightPortType=output  PseudoPeriodic=off  Frequencies=[]  Unit=m  AffineConversion=off
  Sensor_Posicao_peD : sm_lib/Frames and Transforms/Transform Sensor  MeasurementFrame=Base  SenseAngle=off  SenseAxis=off  SenseAngle1=off  SenseAngle2=off  SenseAngle3=off  SenseQ=off  SenseR=off  SenseOmegaX=off  SenseOmegaY=off  SenseOmegaZ=off  SenseOmega1=off  SenseOmega2=off  SenseOmega3=off  SenseQDot=off  SenseRDot=off  SenseAlphaX=off  SenseAlphaY=off  SenseAlphaZ=off  SenseAlpha1=off  SenseAlpha2=off  SenseAlpha3=off  SenseQDDot=off  SenseRDDot=off  SenseX=on  SenseY=on  SenseZ=on  SenseRad=off  SenseAzim=off  SenseDist=off  SenseInc=off  SenseXDot=on  SenseYDot=on  SenseZDot=on  SenseRadDot=off  SenseAzimDot=off  SenseDistDot=off  SenseIncDot=off  SenseXDDot=off  SenseYDDot=off  SenseZDDot=off  SenseRadDDot=off  SenseAzimDDot=off  SenseDistDDot=off  SenseIncDDot=off
  BPD : PMIOPort  Side=Left
  FPD : PMIOPort  Port=2  Side=Left
  pos_peD : Outport
  vel_peD : Outport  Port=2
  wires:
  PS-Simulink Converter7/1 -> Bus Creator1/2  "y"
  PS-Simulink Converter6/1 -> Bus Creator1/1  "x"
  PS-Simulink Converter8/1 -> Bus Creator1/3  "z"
  Bus Creator1/1 -> pos_peD/1
  PS-Simulink Converter1/1 -> Bus Creator/1  "vx"
  PS-Simulink Converter2/1 -> Bus Creator/2  "vy"
  PS-Simulink Converter3/1 -> Bus Creator/3  "vz"
  Bus Creator/1 -> vel_peD/1
  connections:
  Sensor_Posicao_peD/RConn4 -- PS-Simulink Converter8/LConn1
  Sensor_Posicao_peD/RConn3 -- PS-Simulink Converter7/LConn1
  Sensor_Posicao_peD/RConn2 -- PS-Simulink Converter6/LConn1
  BPD/RConn1 -- Sensor_Posicao_peD/LConn1
  Sensor_Posicao_peD/RConn1 -- FPD/RConn1
  PS-Simulink Converter1/LConn1 -- Sensor_Posicao_peD/RConn5
  PS-Simulink Converter2/LConn1 -- Sensor_Posicao_peD/RConn6
  PS-Simulink Converter3/LConn1 -- Sensor_Posicao_peD/RConn7

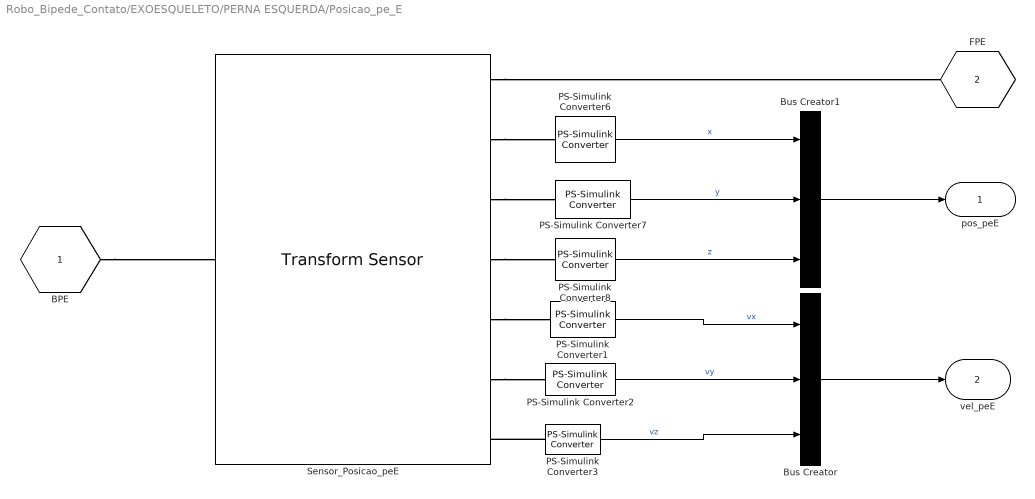
== system Robo_Bipede_Contato/EXOESQUELETO/PERNA ESQUERDA/Posicao_pe_E ==
  Bus Creator : BusCreator  Inputs=3
  Bus Creator1 : BusCreator  Inputs=3
  PS-Simulink Converter1 : nesl_utility/PS-Simulink Converter  PhysicalDomain=network_engine_domain  SubClassName=ps_output  LeftPortType=input  RightPortType=output  PseudoPeriodic=off  Frequencies=[]  Unit=m/s  AffineConversion=off
  PS-Simulink Converter2 : nesl_utility/PS-Simulink Converter  PhysicalDomain=network_engine_domain  SubClassName=ps_output  LeftPortType=input  RightPortType=output  PseudoPeriodic=off  Frequencies=[]  Unit=m/s  AffineConversion=off
  PS-Simulink Converter3 : nesl_utility/PS-Simulink Converter  PhysicalDomain=network_engine_domain  SubClassName=ps_output  LeftPortType=input  RightPortType=output  PseudoPeriodic=off  Frequencies=[]  Unit=m/s  AffineConversion=off
  PS-Simulink Converter6 : nesl_utility/PS-Simulink Converter  PhysicalDomain=network_engine_domain  SubClassName=ps_output  LeftPortType=input  RightPortType=output  PseudoPeriodic=off  Frequencies=[]  Unit=m  AffineConversion=off
  PS-Simulink Converter7 : nesl_utility/PS-Simulink Converter  PhysicalDomain=network_engine_domain  SubClassName=ps_output  LeftPortType=input  RightPortType=output  PseudoPeriodic=off  Frequencies=[]  Unit=m  AffineConversion=off
  PS-Simulink Converter8 : nesl_utility/PS-Simulink Converter  PhysicalDomain=network_engine_domain  SubClassName=ps_output  LeftPortType=input  RightPortType=output  PseudoPeriodic=off  Frequencies=[]  Unit=m  AffineConversion=off
  Sensor_Posicao_peE : sm_lib/Frames and Transforms/Transform Sensor  MeasurementFrame=Base  SenseAngle=off  SenseAxis=off  SenseAngle1=off  SenseAngle2=off  SenseAngle3=off  SenseQ=off  SenseR=off  SenseOmegaX=off  SenseOmegaY=off  SenseOmegaZ=off  SenseOmega1=off  SenseOmega2=off  SenseOmega3=off  SenseQDot=off  SenseRDot=off  SenseAlphaX=off  SenseAlphaY=off  SenseAlphaZ=off  SenseAlpha1=off  SenseAlpha2=off  SenseAlpha3=off  SenseQDDot=off  SenseRDDot=off  SenseX=on  SenseY=on  SenseZ=on  SenseRad=off  SenseAzim=off  SenseDist=off  SenseInc=off  SenseXDot=on  SenseYDot=on  SenseZDot=on  SenseRadDot=off  SenseAzimDot=off  SenseDistDot=off  SenseIncDot=off  SenseXDDot=off  SenseYDDot=off  SenseZDDot=off  SenseRadDDot=off  SenseAzimDDot=off  SenseDistDDot=off  SenseIncDDot=off
  BPE : PMIOPort  Side=Left
  FPE : PMIOPort  Port=2  Side=Left
  pos_peE : Outport
  vel_peE : Outport  Port=2
  wires:
  PS-Simulink Converter7/1 -> Bus Creator1/2  "y"
  PS-Simulink Converter6/1 -> Bus Creator1/1  "x"
  PS-Simulink Converter8/1 -> Bus Creator1/3  "z"
  Bus Creator1/1 -> pos_peE/1
  PS-Simulink Converter1/1 -> Bus Creator/1  "vx"
  PS-Simulink Converter3/1 -> Bus Creator/3  "vz"
  PS-Simulink Converter2/1 -> Bus Creator/2  "vy"
  Bus Creator/1 -> vel_peE/1
  connections:
  Sensor_Posicao_peE/RConn4 -- PS-Simulink Converter8/LConn1
  BPE/RConn1 -- Sensor_Posicao_peE/LConn1
  Sensor_Posicao_peE/RConn3 -- PS-Simulink Converter7/LConn1
  Sensor_Posicao_peE/RConn1 -- FPE/RConn1
  Sensor_Posicao_peE/RConn2 -- PS-Simulink Converter6/LConn1
  PS-Simulink Converter3/LConn1 -- Sensor_Posicao_peE/RConn7
  Sensor_Posicao_peE/RConn5 -- PS-Simulink Converter1/LConn1
  Sensor_Posicao_peE/RConn6 -- PS-Simulink Converter2/LConn1

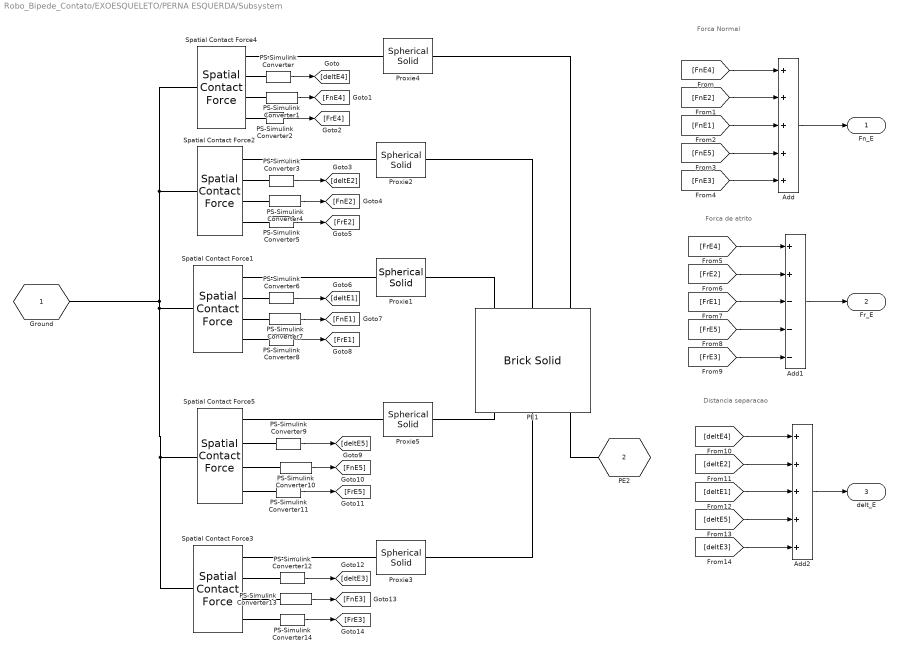
== system Robo_Bipede_Contato/EXOESQUELETO/PERNA ESQUERDA/Subsystem ==
  note: Distancia separacao
  note: Forca de atrito
  note: Forca Normal
  Add : Sum  Inputs=+++++
  Add1 : Sum  Inputs=++---
  Add2 : Sum  Inputs=+++++
  PE1 : sm_lib/Body Elements/Brick Solid  GraphicAmbientColor=[0.15 0.15 0.15 1.0]  BasedOnType=Density  BrickDimensions=[PE.Comprimento, PE.Profundidade, PE.Largura]  BrickDimensionUnits=m  CenterOfMass=[0 0 0]  CenterOfMassUnits=m  GraphicDiffuseColor=cor_pe  Density=rho_ABS  DensityUnits=kg/m^3  DoExposeReferenceFrame=on  GraphicEmissiveColor=[0.0 0.0 0.0 1.0]  ExportEntireGeometry=off  SerializedFrames=<Frames><Frame><Id>Frame1</Id><Value><Name>F1</Name><Origin><Source>GeometricFeature</Source><FeatureName>+z -x curve</FeatureName></Origin><PrimaryAxis><DefinedDirection>+Z</DefinedDirection><Source>ReferenceFrame</Source><SourceDirection>+Z</SourceDirection><FeatureName></FeatureName></PrimaryAxis><SecondaryAxis><DefinedDirection>+X</DefinedDirection><Source>ReferenceFrame</Source><SourceDirection>+X</SourceDirection><FeatureName></FeatureName></SecondaryAxis></Value></Frame><Frame><Id>Frame2</Id><Value><Name>F2</Name><Origin><Source>GeometricFeature</Source><FeatureName>+z +x curve</FeatureName></Origin><PrimaryAxis><DefinedDirection>+Z</DefinedDirection><Source>ReferenceFrame</Source><SourceDirection>+Z</SourceDirection><FeatureName></FeatureName></PrimaryAxis><SecondaryAxis><DefinedDirection>+X</DefinedDirection><Source>ReferenceFrame</Source><SourceDirection>+X</SourceDirection><FeatureName></FeatureName></SecondaryAxis></Value></Frame><Frame><Id>Frame3</Id><Value><Name>F3</Name><Origin><Source>GeometricFeature</Source><FeatureName>-z -x curve</FeatureName></Origin><PrimaryAxis><DefinedDirection>+Z</DefinedDirection><Source>ReferenceFrame</Source><SourceDirection>+Z</SourceDirection><FeatureName></FeatureName></PrimaryAxis><SecondaryAxis><DefinedDirection>+X</DefinedDirection><Source>ReferenceFrame</Source><SourceDirection>+X</SourceDirection><FeatureName></FeatureName></SecondaryAxis></Value></Frame><Frame><Id>Frame4</Id><Value><Name>F4</Name><Origin><Source>GeometricFeature</Source><FeatureName>-z +x curve</FeatureName></Origin><PrimaryAxis><DefinedDirection>+Z</DefinedDirection><Source>ReferenceFrame</Source><SourceDirection>+Z</SourceDirection><FeatureName></FeatureName></PrimaryAxis><SecondaryAxis><DefinedDirection>+X</DefinedDirection><Source>ReferenceFrame</Source><SourceDirection>+X</SourceDirection><FeatureName></FeatureName></SecondaryAxis></Value></Frame><Frame><Id>Frame5</Id><Value><Name>Sup_Pe</Name><Origin><Source>GeometricFeature</Source><FeatureName>+y surface</FeatureName></Origin><PrimaryAxis><DefinedDirection>+Y</DefinedDirection><Source>ReferenceFrame</Source><SourceDirection>+Y</SourceDirection><FeatureName></FeatureName></PrimaryAxis><SecondaryAxis><DefinedDirection>+X</DefinedDirection><Source>ReferenceFrame</Source><SourceDirection>+X</SourceDirection><FeatureName></FeatureName></SecondaryAxis></Value></Frame></Frames>  MarkerShape=Sphere  MarkerSize=10  GraphicType=FromGeometry  InertiaType=CalculateFromGeometry  Mass=1  MassUnits=kg  MomentsOfInertia=[1 1 1]  MomentsOfInertiaUnits=kg*m^2  GraphicOpacity=1.0  ProductsOfInertia=[0 0 0]  ProductsOfInertiaUnits=kg*m^2  GraphicShininess=75  GraphicSpecularColor=[0.5 0.5 0.5 1.0]  GraphicVisPropType=SimpleVisualProperties
  PS-Simulink Converter{,1..14} (15 alike) : nesl_utility/PS-Simulink Converter  PhysicalDomain=network_engine_domain  SubClassName=ps_output  LeftPortType=input  RightPortType=output  PseudoPeriodic=off  Frequencies=[]  Unit=inherit  AffineConversion=off
  Proxie{1..5} (5 alike) : sm_lib/Body Elements/Spherical Solid  GraphicAmbientColor=[0.15 0.15 0.15 1.0]  BasedOnType=Mass  CenterOfMass=[0 0 0]  CenterOfMassUnits=m  GraphicDiffuseColor=[0.5 0.5 0.5]  Density=rho_ABS  DensityUnits=kg/m^3  DoExposeReferenceFrame=on  GraphicEmissiveColor=[0.0 0.0 0.0 1.0]  ExportEntireGeometry=on  SerializedExposedGeometries=<ExposedGeometries><ExposedGeometry><RawGeometryId>entire</RawGeometryId><ExposedGeometryId>G</ExposedGeometryId></ExposedGeometry></ExposedGeometries>  SerializedFrames=<Frames/>  MarkerShape=Sphere  MarkerSize=10  GraphicType=FromGeometry  InertiaType=CalculateFromGeometry  Mass=m_esfera  MassUnits=g  MomentsOfInertia=[1 1 1]  MomentsOfInertiaUnits=kg*m^2  GraphicOpacity=1.0  ProductsOfInertia=[0 0 0]  ProductsOfInertiaUnits=kg*m^2  GraphicShininess=75  GraphicSpecularColor=[0.5 0.5 0.5 1.0]  SphereRadius=PE.Profundidade/2  SphereRadiusUnits=m  GraphicVisPropType=SimpleVisualProperties
  Spatial Contact Force{1..5} (5 alike) : sm_lib/Forces and Torques/Spatial Contact Force  CoefficientOfDynamicFriction=mu_k  CoefficientOfStaticFriction=mu_s  NormalDamping=contact_damping  NormalDampingUnits=N/(m/s)  NormalStiffness=contact_stiffness  NormalStiffnessUnits=N/m  FrictionalCriticalVelocity=mu_vth  FrictionalCriticalVelocityUnits=m/s  ZeroCrossDetectContactStartAndEnd=off  SenseFrictionalForceMagnitude=on  SenseNormalForceMagnitude=on  SenseSeparationDistance=on  NormalTransitionRegionWidth=transition_width  NormalTransitionRegionWidthUnits=m  FrictionType=SmoothStickSlip
  Ground : PMIOPort  Side=Left
  PE2 : PMIOPort  Port=2  Side=Right
  Fn_E : Outport
  Fr_E : Outport  Port=2
  delt_E : Outport  Port=3
  wires:
  PS-Simulink Converter/1 -> [deltE4]
  PS-Simulink Converter1/1 -> [FnE4]
  PS-Simulink Converter2/1 -> [FrE4]
  PS-Simulink Converter5/1 -> [FrE2]
  PS-Simulink Converter4/1 -> [FnE2]
  PS-Simulink Converter3/1 -> [deltE2]
  PS-Simulink Converter7/1 -> [FnE1]
  PS-Simulink Converter6/1 -> [deltE1]
  PS-Simulink Converter8/1 -> [FrE1]
  PS-Simulink Converter10/1 -> [FnE5]
  PS-Simulink Converter9/1 -> [deltE5]
  PS-Simulink Converter11/1 -> [FrE5]
  PS-Simulink Converter13/1 -> [FnE3]
  PS-Simulink Converter12/1 -> [deltE3]
  PS-Simulink Converter14/1 -> [FrE3]
  [FnE4] -> Add/1
  [FnE2] -> Add/2
  [FnE1] -> Add/3
  [FnE5] -> Add/4
  [FnE3] -> Add/5
  [FrE4] -> Add1/1
  [FrE2] -> Add1/2
  [FrE3] -> Add1/5
  [FrE1] -> Add1/3
  [FrE5] -> Add1/4
  [deltE4] -> Add2/1
  [deltE2] -> Add2/2
  [deltE3] -> Add2/5
  [deltE1] -> Add2/3
  [deltE5] -> Add2/4
  Add/1 -> Fn_E/1
  Add1/1 -> Fr_E/1
  Add2/1 -> delt_E/1
  connections:
  Spatial Contact Force4/LConn1 -- Spatial Contact Force3/LConn1 -- Spatial Contact Force5/LConn1 -- Spatial Contact Force1/LConn1 -- Ground/RConn1 -- Spatial Contact Force2/LConn1
  Proxie1/RConn1 -- PE1/LConn1
  Spatial Contact Force4/RConn1 -- Proxie4/LConn1
  Proxie4/RConn1 -- PE1/LConn3
  Spatial Contact Force5/RConn1 -- Proxie5/LConn1
  Spatial Contact Force2/RConn1 -- Proxie2/LConn1
  Spatial Contact Force1/RConn1 -- Proxie1/LConn1
  Proxie5/RConn1 -- PE1/RConn1
  Spatial Contact Force3/RConn1 -- Proxie3/LConn1
  Proxie3/RConn1 -- PE1/RConn2
  Proxie2/RConn1 -- PE1/LConn2
  PE2/RConn1 -- PE1/RConn3
  PS-Simulink Converter/LConn1 -- Spatial Contact Force4/RConn2
  PS-Simulink Converter1/LConn1 -- Spatial Contact Force4/RConn3
  PS-Simulink Converter2/LConn1 -- Spatial Contact Force4/RConn4
  Spatial Contact Force2/RConn4 -- PS-Simulink Converter5/LConn1
  PS-Simulink Converter3/LConn1 -- Spatial Contact Force2/RConn2
  Spatial Contact Force2/RConn3 -- PS-Simulink Converter4/LConn1
  PS-Simulink Converter6/LConn1 -- Spatial Contact Force1/RConn2
  PS-Simulink Converter8/LConn1 -- Spatial Contact Force1/RConn4
  Spatial Contact Force1/RConn3 -- PS-Simulink Converter7/LConn1
  PS-Simulink Converter9/LConn1 -- Spatial Contact Force5/RConn2
  PS-Simulink Converter11/LConn1 -- Spatial Contact Force5/RConn4
  PS-Simulink Converter10/LConn1 -- Spatial Contact Force5/RConn3
  PS-Simulink Converter12/LConn1 -- Spatial Contact Force3/RConn2
  PS-Simulink Converter14/LConn1 -- Spatial Contact Force3/RConn4
  PS-Simulink Converter13/LConn1 -- Spatial Contact Force3/RConn3

== matlab function Robo_Bipede_Contato/EXOESQUELETO/selecionaTorques ==
  settings: updateMethod=DISCRETE
  data: velocidade input; torqueV1 output; torque_dir input; torque_esq input; torqueV2 output; torqueV3 output; torqueV4 output
function [torqueV1,torqueV2,torqueV3,torqueV4] = save_torque(velocidade,torque_dir,torque_esq)

% Seleciona a Struct Data para salvar os torques calculados para as juntas
% da perna direita e da perna esquerda

persistent v
persistent tv1
persistent tv2
persistent tv3
persistent tv4

  
if isempty(v)
    v = velocidade;

    % Constroi as matrizes tipo Persistent para salvar os torques
    % calculados
%     tv1 = zeros(1,length(torque_dir)+length(torque_esq));
%     tv2 = zeros(1,length(torque_dir)+length(torque_esq));
%     tv3 = zeros(1,length(torque_dir)+length(torque_esq));
%     tv4 = zeros(1,length(torque_dir)+length(torque_esq));
     tv1 = zeros(length(torque_dir)+length(torque_esq), 1);
     tv2 = zeros(length(torque_dir)+length(torque_esq), 1);
     tv3 = zeros(length(torque_dir)+length(torque_esq), 1);
     tv4 = zeros(length(torque_dir)+length(torque_esq), 1);
end

% Dependendo da velocidade selecionada, salva os torques das juntas
% switch v
%     case 1
%         tv1 = [torque_dir', torque_esq'];
%                         
%      case 2
%          tv2 = [torque_dir', torque_esq'];
%           
%      case 3
%           tv3 = [torque_dir', torque_esq'];
%                
%      case 4
%           tv4 = [torque_dir', torque_esq'];
% end

    switch v
        case 1
            tv1 = [torque_dir; torque_esq];

         case 2
            tv2 = [torque_dir; torque_esq];

         case 3
            tv3 = [torque_dir; torque_esq];

         case 4
            tv4 = [torque_dir; torque_esq];
    end

v = velocidade;
torqueV1 = tv1;
torqueV2 = tv2;
torqueV3 = tv3;
torqueV4 = tv4;

end
